simulink model "lab6bsim"  (R2023a)
settings: Solver=FixedStepAuto  StartTime=0.0  StopTime=10.0  FixedStep=10/(1024*32)  RelTol=1e-3
undefined symbols (not defined in the file or in its folder): DiscIntNeverNeededParam, lutdata, lutix
settings Model: Creator=andjog  LastModifiedBy=Adde
settings OptimizationCC: ReuseModelBlockBuffer=off

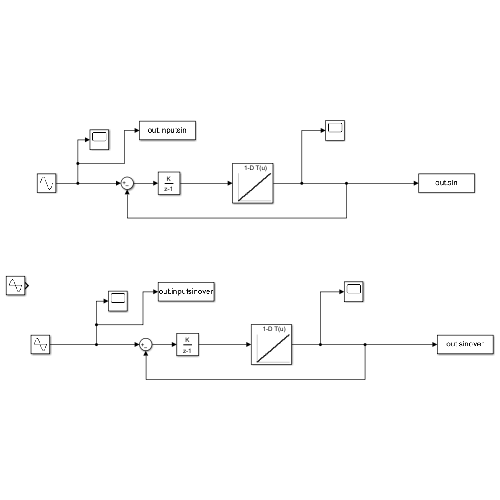
[thumbnail: Simulink's stored preview of the top-level diagram]
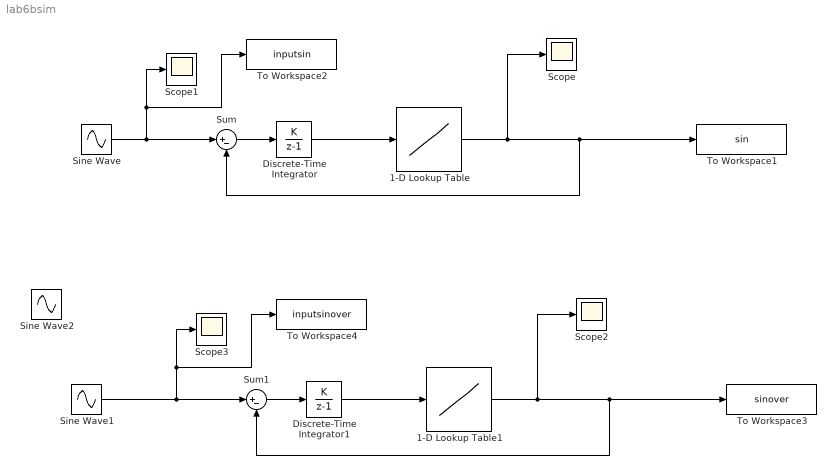
== system lab6bsim ==
  1-D Lookup Table : Lookup_n-D  NumberOfTableDimensions=1  BreakpointsForDimension1=lutix(2^7)  Table=lutdata(2^7)  InternalRulePriority=Speed  RndMeth=Simplest
  1-D Lookup Table1 : Lookup_n-D  NumberOfTableDimensions=1  BreakpointsForDimension1=lutix(2^7)  Table=lutdata(2^7)  InternalRulePriority=Speed  RndMeth=Simplest
  Discrete-Time Integrator : DiscreteIntegrator  IntegratorMethod=Accumulation: Forward Euler  SampleTime=-1  ICPrevOutput=DiscIntNeverNeededParam  ICPrevScaledInput=DiscIntNeverNeededParam
  Discrete-Time Integrator1 : DiscreteIntegrator  IntegratorMethod=Accumulation: Forward Euler  SampleTime=-1  ICPrevOutput=DiscIntNeverNeededParam  ICPrevScaledInput=DiscIntNeverNeededParam
  Scope{,1..3} (4 alike) : Scope
  Sine Wave : Sin  Frequency=pi  SampleTime=0
  Sine Wave1 : Sin  Amplitude=0.88888888  Frequency=pi  SampleTime=0
  Sine Wave2 : Sin  Amplitude=0.8888888  Frequency=pi  SampleTime=0
  Sum : Sum  Inputs=|+-
  Sum1 : Sum  Inputs=|+-
  To Workspace1 : ToWorkspace  VariableName=sin  SaveFormat=Structure With Time  SampleTime=-1
  To Workspace2 : ToWorkspace  VariableName=inputsin  SaveFormat=Structure With Time  SampleTime=-1
  To Workspace3 : ToWorkspace  VariableName=sinover  SaveFormat=Structure With Time  SampleTime=-1
  To Workspace4 : ToWorkspace  VariableName=inputsinover  SaveFormat=Structure With Time  SampleTime=-1
  wires:
  1-D Lookup Table/1 -> To Workspace1/1, Sum/2, Scope/1
  Sine Wave/1 -> To Workspace2/1, Scope1/1, Sum/1
  Sum/1 -> Discrete-Time Integrator/1
  Discrete-Time Integrator/1 -> 1-D Lookup Table/1
  Sine Wave1/1 -> To Workspace4/1, Scope3/1, Sum1/1
  1-D Lookup Table1/1 -> To Workspace3/1, Sum1/2, Scope2/1
  Discrete-Time Integrator1/1 -> 1-D Lookup Table1/1
  Sum1/1 -> Discrete-Time Integrator1/1
